simulink model "MOS2_UE05"  (R2022b)
settings: Solver=ode4  StartTime=0.0  StopTime=100  FixedStep=0.001  RelTol=1e-3
settings Model: Creator=basti  LastModifiedBy=basti

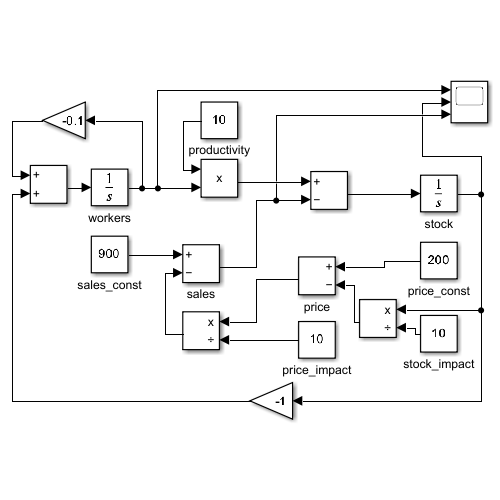
[thumbnail: Simulink's stored preview of the top-level diagram]
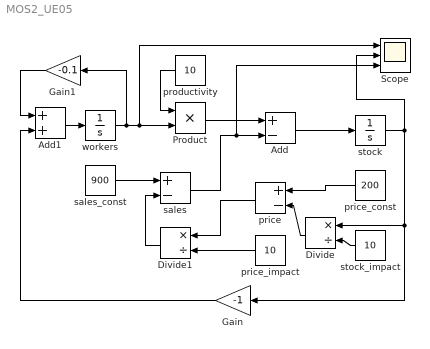
== system MOS2_UE05 ==
  Add : Sum  Inputs=+-
  Add1 : Sum
  Divide : Product  Inputs=*/
  Divide1 : Product  Inputs=*/
  Gain : Gain  Gain=-1
  Gain1 : Gain  Gain=-0.1
  Product : Product
  Scope : Scope  NumInputPorts=3
  price : Sum  Inputs=+-
  price_const : Constant  Value=200
  price_impact : Constant  Value=10
  productivity : Constant  Value=10
  sales : Sum  Inputs=+-
  sales_const : Constant  Value=900
  stock : Integrator  InitialCondition=100
  stock_impact : Constant  Value=10
  workers : Integrator  InitialCondition=50
  wires:
  workers/1 -> Gain1/1, Scope/1, Product/2
  productivity/1 -> Product/1
  Product/1 -> Add/1
  Add/1 -> stock/1
  stock/1 -> Gain/1, Divide/1, Scope/2
  price_const/1 -> price/1
  Divide/1 -> price/2
  stock_impact/1 -> Divide/2
  sales_const/1 -> sales/1
  price_impact/1 -> Divide1/2
  price/1 -> Divide1/1
  Divide1/1 -> sales/2
  sales/1 -> Scope/3, Add/2
  Gain/1 -> Add1/2
  Add1/1 -> workers/1
  Gain1/1 -> Add1/1
